simulink model "Lab_6"  (R2020b)
settings: Solver=VariableStepAuto  StartTime=0.0  StopTime=10.0  RelTol=1e-3
values from neighbouring files (symbols this model uses):
  l1 = input('Link Length 1 : ')    [Lab_10.m]    (also in Lab_11.m = input("link length 1 : "))
  l2 = input('Link Length 2 : ')    [Lab_10.m]    (also in Lab_11.m = input("link length 2: "))
settings Model: Creator=Ghost  LastModifiedBy=Ghost

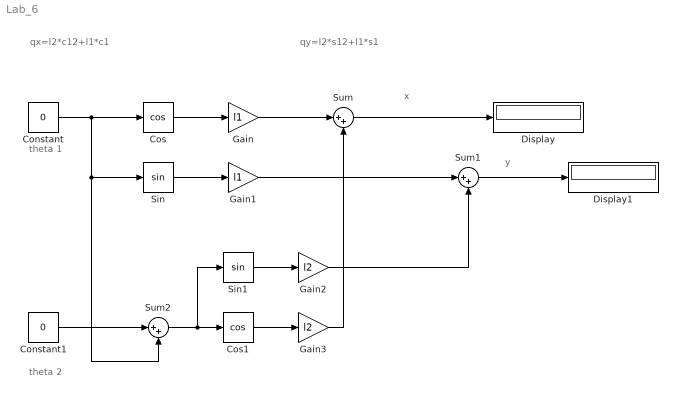
== system Lab_6 ==
  note: qx=l2*c12+l1*c1
  note: y
  note: x
  note: theta 1
  note: theta 2
  note: qy=l2*s12+l1*s1
  Constant : Constant  Value=0
  Constant1 : Constant  Value=0
  Cos : Trigonometry  Operator=cos
  Cos1 : Trigonometry  Operator=cos
  Display : Display
  Display1 : Display
  Gain : Gain  Gain=l1
  Gain1 : Gain  Gain=l1
  Gain2 : Gain  Gain=l2
  Gain3 : Gain  Gain=l2
  Sin : Trigonometry
  Sin1 : Trigonometry
  Sum : Sum  Inputs=|++
  Sum1 : Sum  Inputs=|++
  Sum2 : Sum  Inputs=|++
  wires:
  Constant/1 -> Sum2/2, Sin/1, Cos/1
  Cos/1 -> Gain/1
  Sin/1 -> Gain1/1
  Gain/1 -> Sum/1
  Gain1/1 -> Sum1/1
  Constant1/1 -> Sum2/1
  Sum/1 -> Display/1
  Sum1/1 -> Display1/1
  Sum2/1 -> Sin1/1, Cos1/1
  Sin1/1 -> Gain2/1
  Cos1/1 -> Gain3/1
  Gain3/1 -> Sum/2
  Gain2/1 -> Sum1/2
